simulink library "highFreqFlowData_ul"  (R2018b)
settings: Solver=VariableStepAuto  StartTime=0.0  StopTime=10.0  RelTol=1e-3
libraries: lowFreqFlowData_ul x3
settings Model: Creator=jcreed2  LastModifiedBy=jcreed2

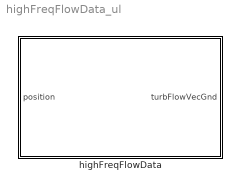
== system highFreqFlowData_ul ==
  highFreqFlowData : Subsystem  mask{flw=0, hFlw=0}
      mask prompts: flw "Low Frequency Flow Obj."; hFlw "High Frequency Flow Obj."

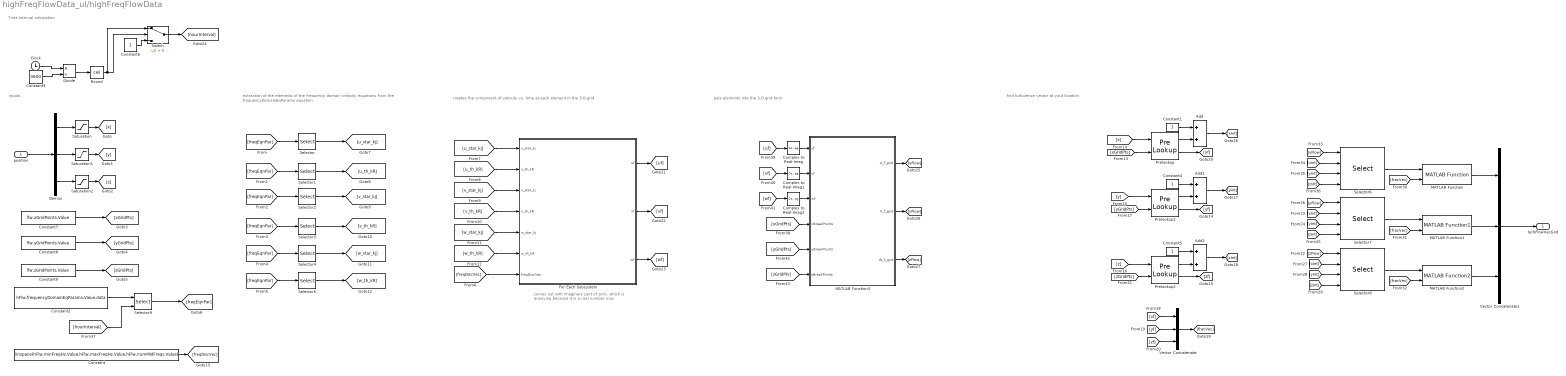
== system highFreqFlowData_ul/highFreqFlowData ==
  note: comes out with imaginary part of zero, which is
      | annoying because it is a real number now
  note: Time Interval calculation
  note: find turbulence vector at yout location
  note: puts elements into the 3-D grid form
  note: extraction of the elements of the frequency domain velocity equations from the
      | frequencyDomainEqParams equation
  note: inputs
  note: creates the component of velocity vs. time at each element in the 3-D grid
  "position " : Inport
  Add : Sum
  Add1 : Sum
  Add2 : Sum
  Clock : Clock
  Complex to Real-Imag : ComplexToRealImag  Output=Real
  Complex to Real-Imag1 : ComplexToRealImag  Output=Real
  Complex to Real-Imag2 : ComplexToRealImag  Output=Real
  Constant : Constant  Value=linspace(hFlw.minFreqHz.Value,hFlw.maxFreqHz.Value,hFlw.numMidFreqs.Value)
  Constant{1,4..6} (4 alike) : Constant
  Constant2 : Constant  Value=hFlw.frequencyDomainEqParams.Value.data
  Constant3 : Constant  Value=3600
  Constant7 : Constant  Value=flw.xGridPoints.Value
  Constant8 : Constant  Value=flw.yGridPoints.Value
  Constant9 : Constant  Value=flw.zGridPoints.Value
  Demux : Demux  Outputs=3
  Divide : Product  Inputs=*/
  For Each Subsystem : Subsystem  TreatAsAtomicUnit=on
  MATLAB Function : lowFreqFlowData_ul/lowFreqFlowData/MATLAB Function  SystemSampleTime=-1
  MATLAB Function1 : lowFreqFlowData_ul/lowFreqFlowData/MATLAB Function1  SystemSampleTime=-1
  MATLAB Function2 : lowFreqFlowData_ul/lowFreqFlowData/MATLAB Function2  SystemSampleTime=-1
  MATLAB Function3 : MATLAB Function  TreatAsAtomicUnit=on
  Prelookup : PreLookup  BreakpointsDataSource=Input port  BreakpointsData=[10:10:110]  BeginIndexSearchUsingPreviousIndexResult=on  ExtrapMethod=Linear
      settings: InputPortMap=u0,p1
  Prelookup1 : PreLookup  BreakpointsDataSource=Input port  BreakpointsData=[10:10:110]  BeginIndexSearchUsingPreviousIndexResult=on  ExtrapMethod=Linear
      settings: InputPortMap=u0,p1
  Prelookup2 : PreLookup  BreakpointsDataSource=Input port  BreakpointsData=[10:10:110]  BeginIndexSearchUsingPreviousIndexResult=on  ExtrapMethod=Linear
      settings: InputPortMap=u0,p1
  Round : Rounding  Operator=ceil
  Saturation : Saturate
  Saturation1 : Saturate
  Saturation2 : Saturate
  Selector : Selector  NumberOfDimensions=3  InputPortWidth=3  IndexOptions=Select all,Select all,Index vector (dialog)  Indices=[1 3],1,1  OutputSizes=1,1,1
  Selector1 : Selector  NumberOfDimensions=3  InputPortWidth=3  IndexOptions=Select all,Select all,Index vector (dialog)  Indices=[1 3],1,2  OutputSizes=1,1,1
  Selector2 : Selector  NumberOfDimensions=3  InputPortWidth=3  IndexOptions=Select all,Select all,Index vector (dialog)  Indices=[1 3],1,3  OutputSizes=1,1,1
  Selector3 : Selector  NumberOfDimensions=3  InputPortWidth=3  IndexOptions=Select all,Select all,Index vector (dialog)  Indices=[1 3],1,4  OutputSizes=1,1,1
  Selector4 : Selector  NumberOfDimensions=3  InputPortWidth=3  IndexOptions=Select all,Select all,Index vector (dialog)  Indices=[1 3],1,5  OutputSizes=1,1,1
  Selector5 : Selector  NumberOfDimensions=3  InputPortWidth=3  IndexOptions=Select all,Select all,Index vector (dialog)  Indices=[1 3],1,6  OutputSizes=1,1,1
  Selector6 : Selector  NumberOfDimensions=3  InputPortWidth=3  IndexOptions=Starting index (port),Starting index (port),Starting index (port)  Indices=[1 3],1,1  OutputSizes=2,2,2
  Selector7 : Selector  NumberOfDimensions=3  InputPortWidth=3  IndexOptions=Starting index (port),Starting index (port),Starting index (port)  Indices=[1 3],1,1  OutputSizes=2,2,2
  Selector8 : Selector  NumberOfDimensions=3  InputPortWidth=3  IndexOptions=Starting index (port),Starting index (port),Starting index (port)  Indices=[1 3],1,1  OutputSizes=2,2,2
  Selector9 : Selector  NumberOfDimensions=4  InputPortWidth=3  IndexOptions=Select all,Select all,Select all,Starting index (port)  Indices=[1 3],1,1,1  OutputSizes=1,1,1,1
  Switch : Switch  Criteria=u2 > Threshold
  Vector Concatenate : Concatenate  NumInputs=3
  Vector Concatenate1 : Concatenate  NumInputs=3
  turbFlowVecGnd : Outport
  wires:
  Saturation/1 -> [x]
  [freqDiscVec] -> For Each Subsystem/7(freqDiscVec)
  [freqEqnPar] -> Selector2/1
  Demux/2 -> Saturation1/1
  Demux/3 -> Saturation2/1
  [freqEqnPar] -> Selector3/1
  Selector1/1 -> [u_th_kR]
  [w_star_kj] -> For Each Subsystem/5(w_star_kj)
  Constant8/1 -> [yGridPts]
  Constant9/1 -> [zGridPts]
  Selector2/1 -> [v_star_kj]
  [v_star_kj] -> For Each Subsystem/3(v_star_kj)
  [freqEqnPar] -> Selector/1
  Saturation2/1 -> [z]
  [w_th_kR] -> For Each Subsystem/6(w_th_kR)
  Constant7/1 -> [xGridPts]
  [freqEqnPar] -> Selector5/1
  Constant/1 -> [freqDiscVec]
  Selector5/1 -> [w_th_kR]
  [u_th_kR] -> For Each Subsystem/2(u_th_kR)
  [freqEqnPar] -> Selector4/1
  [freqEqnPar] -> Selector1/1
  Selector4/1 -> [w_star_kj]
  [u_star_kj] -> For Each Subsystem/1(u_star_kj)
  Demux/1 -> Saturation/1
  Selector3/1 -> [v_th_kR]
  Saturation1/1 -> [y]
  For Each Subsystem/2(vf) -> [vf]
  [v_th_kR] -> For Each Subsystem/4(v_th_kR)
  For Each Subsystem/1(uf) -> [uf]
  Selector/1 -> [u_star_kj]
  For Each Subsystem/3("wf ") -> [wf]
  [zGridPts] -> Prelookup2/2
  Prelookup2/2 -> [zf]
  Vector Concatenate/1 -> [fracVec]
  [z] -> Prelookup2/1
  [x] -> Prelookup/1
  [yGridPts] -> Prelookup1/2
  [y] -> Prelookup1/1
  [yf] -> Vector Concatenate/2
  [xf] -> Vector Concatenate/1
  [zf] -> Vector Concatenate/3
  Prelookup2/1 -> Add2/2
  Constant5/1 -> Add2/1
  Add2/1 -> [zInt]
  Prelookup1/1 -> Add1/2
  Prelookup/1 -> Add/2
  Constant1/1 -> Add/1
  [xGridPts] -> Prelookup/2
  Add/1 -> [xInt]
  Prelookup1/2 -> [yf]
  Prelookup/2 -> [xf]
  Add1/1 -> [yInt]
  Constant4/1 -> Add1/1
  [yInt] -> Selector6/3
  [fracVec] -> MATLAB Function1/2
  [fracVec] -> MATLAB Function/2
  [fracVec] -> MATLAB Function2/2
  [yInt] -> Selector7/3
  [yInt] -> Selector8/3
  MATLAB Function/1 -> Vector Concatenate1/1
  Selector8/1 -> MATLAB Function2/1
  [zFlow] -> Selector8/1
  [zInt] -> Selector7/4
  [zInt] -> Selector8/4
  MATLAB Function1/1 -> Vector Concatenate1/2
  Selector7/1 -> MATLAB Function1/1
  [yFlow] -> Selector7/1
  [xFlow] -> Selector6/1
  [xInt] -> Selector8/2
  Selector6/1 -> MATLAB Function/1
  [zInt] -> Selector6/4
  MATLAB Function2/1 -> Vector Concatenate1/3
  [xInt] -> Selector6/2
  [xInt] -> Selector7/2
  Round/1 -> Switch/1, Switch/2
  Constant6/1 -> Switch/3
  Switch/1 -> [hourInterval]
  Divide/1 -> Round/1
  Constant3/1 -> Divide/2
  Clock/1 -> Divide/1
  Constant2/1 -> Selector9/1
  Selector9/1 -> [freqEqnPar]
  [hourInterval] -> Selector9/2
  [xGridPts] -> MATLAB Function3/4(xBreakPoints)
  [uf] -> Complex to Real-Imag/1
  [vf] -> Complex to Real-Imag1/1
  [wf] -> Complex to Real-Imag2/1
  [yGridPts] -> MATLAB Function3/5(yBreakPoints)
  [zGridPts] -> MATLAB Function3/6(zBreakPoints)
  MATLAB Function3/1(U_f_grid) -> [xFlow]
  MATLAB Function3/2(V_f_grid) -> [yFlow]
  MATLAB Function3/3(W_f_grid) -> [zFlow]
  Complex to Real-Imag/1 -> MATLAB Function3/1(uf)
  Complex to Real-Imag1/1 -> MATLAB Function3/2(vf)
  Complex to Real-Imag2/1 -> MATLAB Function3/3(wf)
  "position "/1 -> Demux/1
  Vector Concatenate1/1 -> turbFlowVecGnd/1

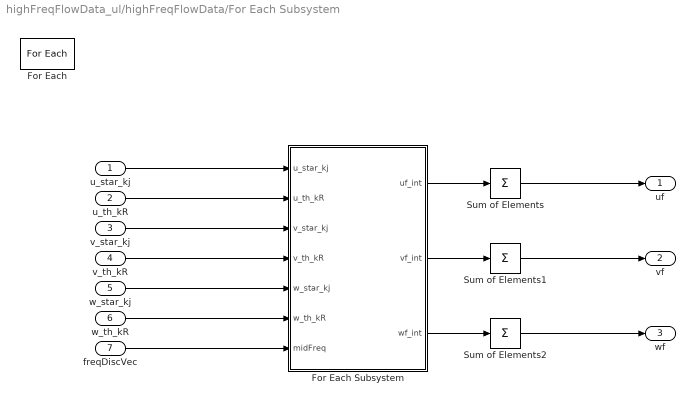
== system highFreqFlowData_ul/highFreqFlowData/For Each Subsystem ==
  u_star_kj : Inport  Partition=on  PartitionDimension=1  PartitionWidth=1  PartitionOffset=0
  u_th_kR : Inport  Port=2  Partition=on  PartitionDimension=1  PartitionWidth=1  PartitionOffset=0
  v_star_kj : Inport  Port=3  Partition=on  PartitionDimension=1  PartitionWidth=1  PartitionOffset=0
  v_th_kR : Inport  Port=4  Partition=on  PartitionDimension=1  PartitionWidth=1  PartitionOffset=0
  w_star_kj : Inport  Port=5  Partition=on  PartitionDimension=1  PartitionWidth=1  PartitionOffset=0
  w_th_kR : Inport  Port=6  Partition=on  PartitionDimension=1  PartitionWidth=1  PartitionOffset=0
  freqDiscVec : Inport  Port=7
  For Each : ForEach  DisableCoverage=on  IndexMode=One-based
  For Each Subsystem : Subsystem  TreatAsAtomicUnit=on
  Sum of Elements : Sum  Inputs=+
  Sum of Elements1 : Sum  Inputs=+
  Sum of Elements2 : Sum  Inputs=+
  uf : Outport  ConcatenationDimension=1
  vf : Outport  Port=2  ConcatenationDimension=1
  "wf " : Outport  Port=3  ConcatenationDimension=1
  wires:
  For Each Subsystem/1(uf_int) -> Sum of Elements/1
  Sum of Elements/1 -> uf/1
  For Each Subsystem/2(vf_int) -> Sum of Elements1/1
  Sum of Elements1/1 -> vf/1
  For Each Subsystem/3("wf_int ") -> Sum of Elements2/1
  Sum of Elements2/1 -> "wf "/1
  u_star_kj/1 -> For Each Subsystem/1(u_star_kj)
  u_th_kR/1 -> For Each Subsystem/2(u_th_kR)
  v_star_kj/1 -> For Each Subsystem/3(v_star_kj)
  v_th_kR/1 -> For Each Subsystem/4(v_th_kR)
  w_star_kj/1 -> For Each Subsystem/5(w_star_kj)
  w_th_kR/1 -> For Each Subsystem/6(w_th_kR)
  freqDiscVec/1 -> For Each Subsystem/7("midFreq ")

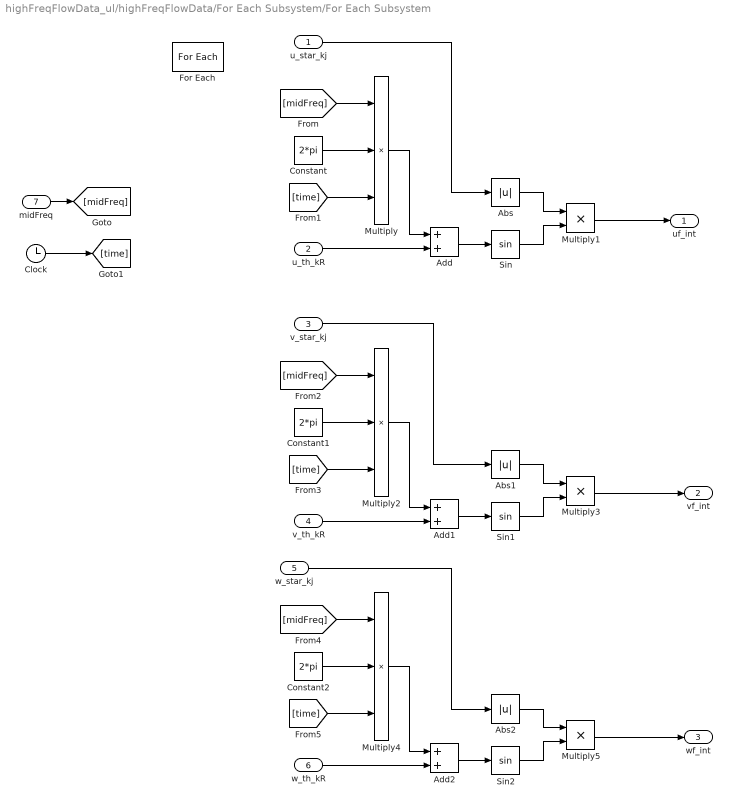
== system highFreqFlowData_ul/highFreqFlowData/For Each Subsystem/For Each Subsystem ==
  u_star_kj : Inport  Partition=on  PartitionDimension=2  PartitionWidth=1  PartitionOffset=0
  u_th_kR : Inport  Port=2  Partition=on  PartitionDimension=2  PartitionWidth=1  PartitionOffset=0
  v_star_kj : Inport  Port=3  Partition=on  PartitionDimension=2  PartitionWidth=1  PartitionOffset=0
  v_th_kR : Inport  Port=4  Partition=on  PartitionDimension=2  PartitionWidth=1  PartitionOffset=0
  w_star_kj : Inport  Port=5  Partition=on  PartitionDimension=2  PartitionWidth=1  PartitionOffset=0
  w_th_kR : Inport  Port=6  Partition=on  PartitionDimension=2  PartitionWidth=1  PartitionOffset=0
  "midFreq " : Inport  Port=7  Partition=on  PartitionDimension=1  PartitionWidth=1  PartitionOffset=0
  Abs : Abs
  Abs1 : Abs
  Abs2 : Abs
  Add : Sum
  Add1 : Sum
  Add2 : Sum
  Clock : Clock
  Constant : Constant  Value=2*pi
  Constant1 : Constant  Value=2*pi
  Constant2 : Constant  Value=2*pi
  For Each : ForEach  DisableCoverage=on  IndexMode=One-based
  Multiply : Product  Inputs=3
  Multiply1 : Product
  Multiply2 : Product  Inputs=3
  Multiply3 : Product
  Multiply4 : Product  Inputs=3
  Multiply5 : Product
  Sin : Trigonometry
  Sin1 : Trigonometry
  Sin2 : Trigonometry
  uf_int : Outport  ConcatenationDimension=2
  vf_int : Outport  Port=2  ConcatenationDimension=2
  "wf_int " : Outport  Port=3  ConcatenationDimension=2
  wires:
  u_star_kj/1 -> Abs/1
  "midFreq "/1 -> [midFreq]
  Clock/1 -> [time]
  [midFreq] -> Multiply/1
  Constant/1 -> Multiply/2
  [time] -> Multiply/3
  Multiply/1 -> Add/1
  u_th_kR/1 -> Add/2
  Add/1 -> Sin/1
  Abs/1 -> Multiply1/1
  Sin/1 -> Multiply1/2
  Multiply1/1 -> uf_int/1
  [midFreq] -> Multiply2/1
  Constant1/1 -> Multiply2/2
  [time] -> Multiply2/3
  Multiply2/1 -> Add1/1
  v_th_kR/1 -> Add1/2
  Add1/1 -> Sin1/1
  v_star_kj/1 -> Abs1/1
  Abs1/1 -> Multiply3/1
  Sin1/1 -> Multiply3/2
  Multiply3/1 -> vf_int/1
  [midFreq] -> Multiply4/1
  Constant2/1 -> Multiply4/2
  [time] -> Multiply4/3
  Multiply4/1 -> Add2/1
  Add2/1 -> Sin2/1
  Abs2/1 -> Multiply5/1
  Sin2/1 -> Multiply5/2
  Multiply5/1 -> "wf_int "/1
  w_th_kR/1 -> Add2/2
  w_star_kj/1 -> Abs2/1

== matlab function highFreqFlowData_ul/highFreqFlowData/MATLAB Function3 ==
  data: uf input; U_f_grid output; vf input; wf input; xBreakPoints input; yBreakPoints input; zBreakPoints input; V_f_grid output; W_f_grid output
function [  U_f_grid,  V_f_grid,  W_f_grid ]= fcn(uf,vf,wf, xBreakPoints,yBreakPoints,zBreakPoints)


xS = size( xBreakPoints );
yS = size( yBreakPoints );
zS = size( zBreakPoints );

n_elem = xS(1)*yS(1)*zS(1);

U_f_grid  = NaN(xS(1),yS(1),zS(1));
V_f_grid  = NaN(xS(1),yS(1),zS(1));
W_f_grid  = NaN(xS(1),yS(1),zS(1));

    for i = 1:n_elem
        
        U_f_grid(i) = uf(i);
        V_f_grid(i) = vf(i);
        W_f_grid(i) = wf(i);
        
    end

end
